simulink model "extended_discrete_kalman_filter"  (R2015b)
settings: Solver=VariableStepAuto  StartTime=0.0  StopTime=10.0  RelTol=1e-3
settings Model: Creator=mgreiff  LastModifiedBy=mgreiff

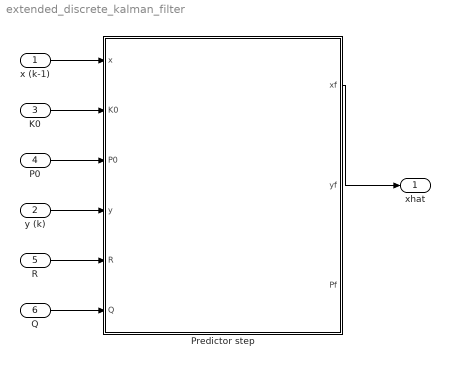
== system extended_discrete_kalman_filter ==
  x (k-1) : Inport  PortDimensions=12
  y (k) : Inport  Port=2  PortDimensions=6
  K0 : Inport  Port=3
  P0 : Inport  Port=4
  R : Inport  Port=5
  Q : Inport  Port=6
  Predictor step : MATLAB Function  TreatAsAtomicUnit=on
  xhat : Outport
  wires:
  Predictor step/1(xf) -> xhat/1
  x (k-1)/1 -> Predictor step/1(x)
  y (k)/1 -> Predictor step/4(y)
  K0/1 -> Predictor step/2(K0)
  P0/1 -> Predictor step/3(P0)
  R/1 -> Predictor step/5(R)
  Q/1 -> Predictor step/6(Q)

== matlab function extended_discrete_kalman_filter/Predictor step ==
  data: x input; K0 input; P0 input; y input; xf output; R input; Q input; yf output; Pf output
function [xf, yf, Pf] = fcn(x, K0, P0, y, R, Q)
%#codegen
persistent P K

if isempty(P)
    P = P0;
    K = K0;
end

%% Set up basic continuous-model dynamics, including PD
Ad = diag(A);
a1 = 4.8; a2 = 8.32; b = 8.32;
a1 = KetaD(1); a2 = KetaP(1); b = KetaP(1);

T0 = m*g;

Am1 = [zeros(10,3)];
Am2 = [eye(3); -Ad/m; zeros(4,3)];
Am3 = [zeros(3,2); T0/m 0; 0 -T0/m; zeros(3,2); -a2*eye(2)];
Am4 = [zeros(6,2); eye(2); -a1*eye(2)];
Am = [Am1 Am2 Am3 Am4];

xf = 1;
yf = 1;
y = 1;

%% Corrector step
xa = xf + K * (y - yf);
Jh = 1; % Evaluate jacobian around xf
K = Pf * J / (J * P * J' + R);
P = (eye(1) - K * Jh) * Pf;
xhat = xa;
